simulink model "TriggeredSubsystem"  (R2020b)
settings: Solver=VariableStepAuto  StartTime=0.0  StopTime=2  MaxStep=0.001  RelTol=1e-3
settings Model: Creator=99003778  LastModifiedBy=99003778

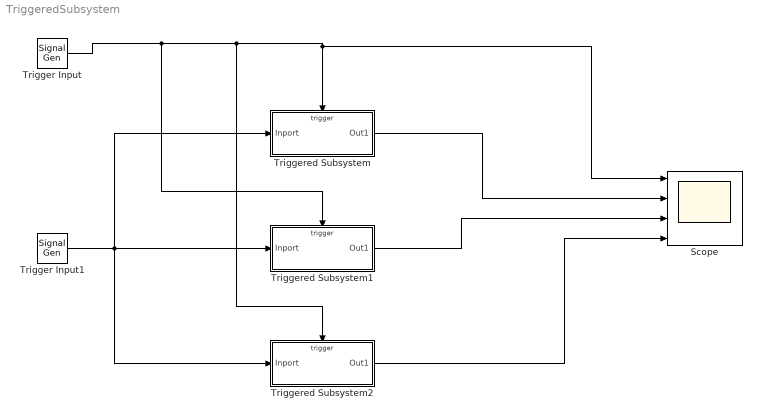
== system TriggeredSubsystem ==
  Scope : Scope  NumInputPorts=4
  Trigger Input : SignalGenerator  WaveForm=square  Frequency=3
  Trigger Input1 : SignalGenerator
  Triggered Subsystem : Subsystem  TreatAsAtomicUnit=on
  Triggered Subsystem1 : Subsystem  TreatAsAtomicUnit=on
  Triggered Subsystem2 : Subsystem  TreatAsAtomicUnit=on
  wires:
  Trigger Input/1 -> Triggered Subsystem1/Trigger, Triggered Subsystem2/Trigger, Triggered Subsystem/Trigger, Scope/1
  Triggered Subsystem/1(Out1) -> Scope/2
  Triggered Subsystem1/1(Out1) -> Scope/3
  Triggered Subsystem2/1(Out1) -> Scope/4
  Trigger Input1/1 -> Triggered Subsystem2/1(Inport), Triggered Subsystem/1(Inport), Triggered Subsystem1/1(Inport)

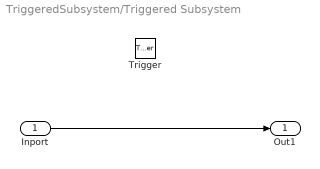
== system TriggeredSubsystem/Triggered Subsystem ==
  Inport : Inport
  Trigger : TriggerPort  VariantControl=Variant
  Out1 : Outport
  wires:
  Inport/1 -> Out1/1

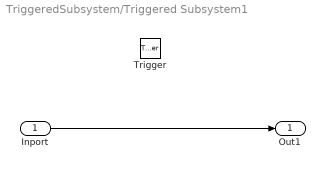
== system TriggeredSubsystem/Triggered Subsystem1 ==
  Inport : Inport
  Trigger : TriggerPort  TriggerType=falling  VariantControl=Variant
  Out1 : Outport
  wires:
  Inport/1 -> Out1/1

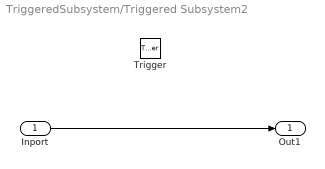
== system TriggeredSubsystem/Triggered Subsystem2 ==
  Inport : Inport
  Trigger : TriggerPort  TriggerType=either  VariantControl=Variant
  Out1 : Outport
  wires:
  Inport/1 -> Out1/1
